simulink model "qd2pwmtest"  (R2016a)
settings: Solver=ode5  StartTime=0.0  StopTime=inf  FixedStep=0.001  RelTol=1e-3
libraries: dcpctrl x1
settings Model: SimulationMode=external  Creator=julianleland  LastModifiedBy=julianleland
settings HardwareCC: ProdBitPerLong=64  ProdLargestAtomicFloat=None  ProdHWDeviceType=Intel->x86-64  TargetBitPerLong=64  TargetBitPerPointer=64  TargetIntDivRoundTo=Zero  TargetEndianess=LittleEndian  TargetWordSize=64  TargetHWDeviceType=Intel->x86-64
settings RTWCC: SystemTargetFile=sldrt.tlc  TemplateMakefile=sldrt.tmf  Description=Simulink Desktop Real-Time  RTWCompilerOptimization=on
settings CodeAppCC: MaxIdLength=95
settings SimulinkDesktopRealTimeCC: TargetPreCompLibLocation=/Applications/MATLAB_R2016a.app/toolbox/sldrt/lib/maci64  TargetLangStandard=C89/C90 (ANSI)  SupportVariableSizeSignals=off

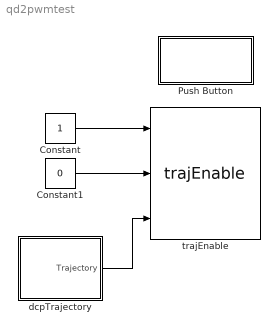
== system qd2pwmtest ==
  Constant : Constant
  Constant1 : Constant  Value=0
  Push Button : Subsystem  DialogController=hmiCreateDDGDialog  IsWebBlock=on  mask(MWDashboardBlock){webBlockId=70571214-1623-4fe4-a991-a5e4601e90b3, webBlockType=pushbutton, ShowInLibBrwoser=on, ShowInitialText=on, HMISrcModelName=qd2pwmtest}
      mask prompts: webBlockId "WebBlock Id"; webBlockType "WebBlock Type"; HMISrcModelName "Source Model"
      mask Help: helpview([docroot '/mapfiles/simulink.map'], 'hmi_push_button')
      mask Display:
      | model = bdroot(gcb);
      | if strcmp(get_param(model,'BlockDiagramType'), 'library')
      |     image([(matlabroot) '/toolbox/simulink/hmi/icons/PushButton.png']);
      | end
  dcpTrajectory : Subsystem
  trajEnable : dcpctrl/trajEnable
  wires:
  dcpTrajectory/1(Trajectory) -> trajEnable/3
  Constant1/1 -> trajEnable/2
  Constant/1 -> trajEnable/1

== system qd2pwmtest/Push Button ==

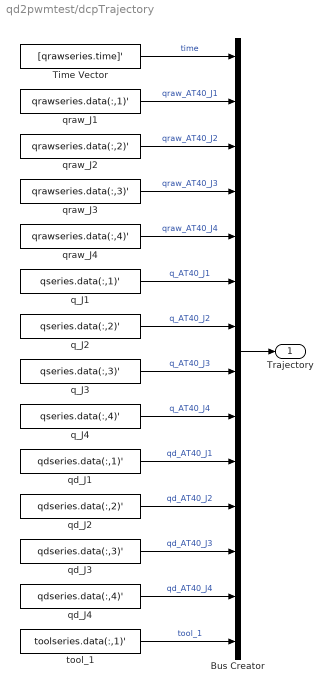
== system qd2pwmtest/dcpTrajectory ==
  Bus Creator : BusCreator  Inputs='time','qraw_AT40_J1','qraw_AT40_J2','qraw_AT40_J3','qraw_AT40_J4','q_AT40_J1','q_AT40_J2','q_AT40_J3','q_AT40_J4','qd_AT40_J1','qd_AT40_J2','qd_AT40_J3','qd_AT40_J4','tool_1'
  Time Vector : FromWorkspace  VariableName=[qrawseries.time]'  SampleTime=0
  q_J1 : FromWorkspace  VariableName=qseries.data(:,1)'  SampleTime=0
  q_J2 : FromWorkspace  VariableName=qseries.data(:,2)'  SampleTime=0
  q_J3 : FromWorkspace  VariableName=qseries.data(:,3)'  SampleTime=0
  q_J4 : FromWorkspace  VariableName=qseries.data(:,4)'  SampleTime=0
  qd_J1 : FromWorkspace  VariableName=qdseries.data(:,1)'  SampleTime=0
  qd_J2 : FromWorkspace  VariableName=qdseries.data(:,2)'  SampleTime=0
  qd_J3 : FromWorkspace  VariableName=qdseries.data(:,3)'  SampleTime=0
  qd_J4 : FromWorkspace  VariableName=qdseries.data(:,4)'  SampleTime=0
  qraw_J1 : FromWorkspace  VariableName=qrawseries.data(:,1)'  SampleTime=0
  qraw_J2 : FromWorkspace  VariableName=qrawseries.data(:,2)'  SampleTime=0
  qraw_J3 : FromWorkspace  VariableName=qrawseries.data(:,3)'  SampleTime=0
  qraw_J4 : FromWorkspace  VariableName=qrawseries.data(:,4)'  SampleTime=0
  tool_1 : FromWorkspace  VariableName=toolseries.data(:,1)'  SampleTime=0
  Trajectory : Outport
  wires:
  tool_1/1 -> Bus Creator/14  "tool_1"
  Bus Creator/1 -> Trajectory/1
  qraw_J4/1 -> Bus Creator/5  "qraw_AT40_J4"
  qraw_J2/1 -> Bus Creator/3  "qraw_AT40_J2"
  Time Vector/1 -> Bus Creator/1  "time"
  qraw_J3/1 -> Bus Creator/4  "qraw_AT40_J3"
  qraw_J1/1 -> Bus Creator/2  "qraw_AT40_J1"
  q_J1/1 -> Bus Creator/6  "q_AT40_J1"
  q_J2/1 -> Bus Creator/7  "q_AT40_J2"
  q_J3/1 -> Bus Creator/8  "q_AT40_J3"
  q_J4/1 -> Bus Creator/9  "q_AT40_J4"
  qd_J1/1 -> Bus Creator/10  "qd_AT40_J1"
  qd_J2/1 -> Bus Creator/11  "qd_AT40_J2"
  qd_J3/1 -> Bus Creator/12  "qd_AT40_J3"
  qd_J4/1 -> Bus Creator/13  "qd_AT40_J4"
